simulink model "speed_to_pulse"  (R2017a)
settings: Solver=VariableStepAuto  StartTime=0.0  StopTime=50000  RelTol=1e-3
libraries: simulink x1, hdlsllib x1
settings Model: Creator=Ryan Corkery  LastModifiedBy=Ryan Corkery

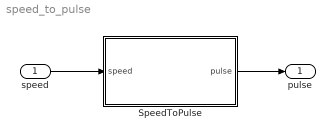
== system speed_to_pulse ==
  speed : Inport  OutDataTypeStr=uint8
  SpeedToPulse : Subsystem
  pulse : Outport
  wires:
  speed/1 -> SpeedToPulse/1(speed)
  SpeedToPulse/1(pulse) -> pulse/1

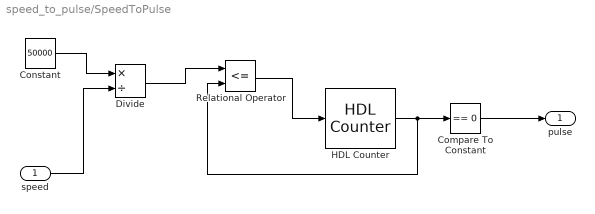
== system speed_to_pulse/SpeedToPulse ==
  speed : Inport  OutDataTypeStr=uint8
  Compare To Constant : simulink/Logic and Bit Operations/Compare To Constant  relop===  const=0  OutDataTypeStr=boolean
  Constant : Constant  Value=50000  OutDataTypeStr=uint32  SampleTime=1
  Divide : Product  Inputs=*/  SaturateOnIntegerOverflow=on  RndMeth=Zero
  HDL Counter : hdlsllib/HDL Operations/HDL Counter  CountType=Free running  CountInit=0  CountStep=1  CountMax=25  CountFromType=Initial value  CountFrom=0  CountResetPort=on  CountLoadPort=off  CountEnbPort=off  CountDirPort=off  CountDataType=Unsigned  CountWordLen=32  CountFracLen=0  CountSampTime=1
      settings: SourceProductName=HDL Coder  SourceProductBaseCode=HD
  Relational Operator : RelationalOperator  Operator=<=  OutDataTypeStr=boolean  RndMeth=Nearest
  pulse : Outport
  wires:
  Divide/1 -> Relational Operator/1
  Compare To Constant/1 -> pulse/1
  HDL Counter/1 -> Relational Operator/2, Compare To Constant/1
  Relational Operator/1 -> HDL Counter/1
  Constant/1 -> Divide/1
  speed/1 -> Divide/2
